simulink model "Model_15_11062020_3_Lev_Unbalance_SVM_AB21"  (R2021a)
settings: Solver=FixedStepAuto  StartTime=0.0  StopTime=0.03  FixedStep=Ts/10  MaxStep=1e-4  RelTol=1e-3
InitFcn:
  | Ts=1/(12000);
  | Ts_Control=Ts;
  | Ts_Power=Ts;
  | PulseDuration=5e-6;
  | Vrefpeak=399;
  | VDC=800;
  | R=1.4;
  | L=1e-4;
  | Freq = 120;
  | Rc= 0.00001;
  | C=220e-6;
  | Ld = 473e-6;
  | Lq = 1155e-6;
  | Fpm = 0.1383;
  | Rs = 0.036;
  | 
  | 
  | %%%%%Switch Characterization START%%%%%
  | T003_Thermal_Initialization;
  | T020_Characterizing_SKiM401MLI07E4_Simulink_Model_v1_0;
  | %%%%%Switch Characterization END%%%%%%
undefined symbols (not defined in the file or in its folder): Cond_Loss_Diode, Cond_Loss_IGBT, Page_Temp_C, Reverse_Rec_Diode, TurnoffIGBT, TurnonIGBT
libraries: spsMeanLib x35, simulink x28, spsMonostableLib x14, spsSampleandHoldLib x14, spsIGBTDiodeLib x12, spsDiodeLib x6, spsCurrentMeasurementLib x4, spsFirstOrderFilterLib x3, spsSeriesRLCBranchLib x3, spsVoltageMeasurementLib x3, pid_lib x2, spsAlphaBetaZerotoabcLib x1
(part 2 of 2)

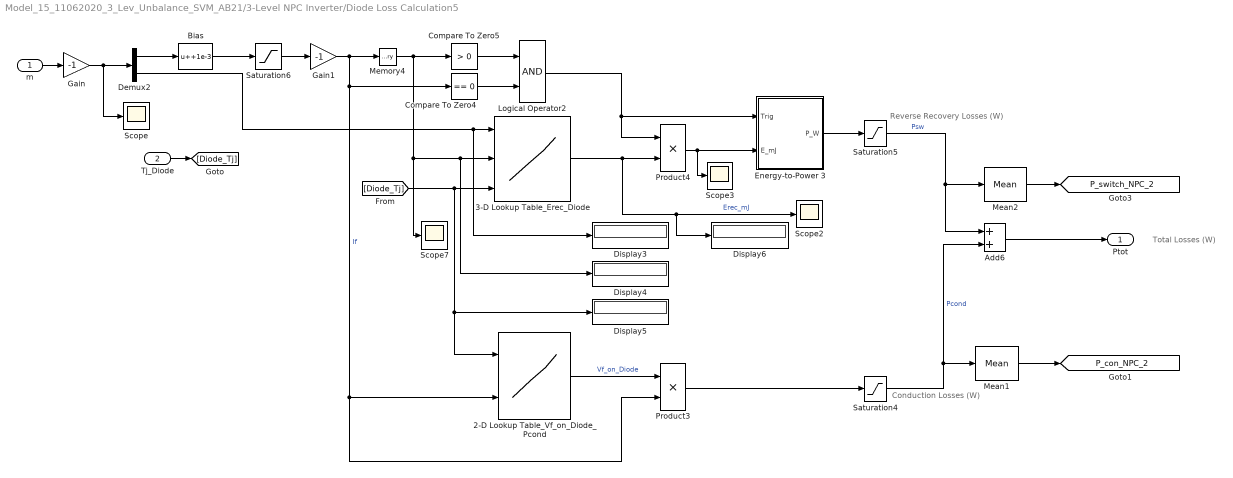
== system Model_15_11062020_3_Lev_Unbalance_SVM_AB21/3-Level NPC Inverter/Diode Loss Calculation5 ==
  note: Conduction Losses (W)
  note: Total Losses (W)
  note: Reverse Recovery Losses (W)
  m : Inport
  Tj_Diode : Inport  Port=2
  2-D Lookup Table_Vf_on_Diode_Pcond : Lookup_n-D  BreakpointsForDimension1=Cond_Loss_Diode.Tj  BreakpointsForDimension2=Cond_Loss_Diode.Ic  BreakpointsForDimension3=Page_Temp_C  Table=Cond_Loss_Diode.Vce  RndMeth=Simplest  InputSameDT=on
      settings: InputPortMap=u0,u1
  3-D Lookup Table_Erec_Diode : Lookup_n-D  NumberOfTableDimensions=3  BreakpointsForDimension1=Reverse_Rec_Diode.Vcc_Esw_Erec  BreakpointsForDimension2=Reverse_Rec_Diode.DIODE_If_Erec  BreakpointsForDimension3=Reverse_Rec_Diode.DIODE_Tj_Erec  Table=Reverse_Rec_Diode.Esw_Erec  RndMeth=Simplest  InputSameDT=on
      settings: InputPortMap=u0,u1,u2
  Add6 : Sum
  Bias : Bias  Bias=+1e-3
  Compare To Zero4 : simulink/Logic and Bit Operations/Compare To Zero  relop===  OutDataTypeStr=boolean
  Compare To Zero5 : simulink/Logic and Bit Operations/Compare To Zero  relop=>  OutDataTypeStr=boolean
  Demux2 : Demux  Outputs=2
  Display{3..6} (4 alike) : Display
  Energy-to-Power 3 : Subsystem  mask{PulseDuration=PulseDuration, Ts=Ts}
      mask prompts: PulseDuration "Pulse Duration (s):"; Ts "Sample time (s):"
  Gain : Gain  Gain=-1
  Gain1 : Gain  Gain=-1
  Logical Operator2 : Logic  AllPortsSameDT=off  OutDataTypeStr=float('double')
  Mean1 : spsMeanLib/Mean  Freq=Freq  Vinit=0  Ts=0
  Mean2 : spsMeanLib/Mean  Freq=Freq  Vinit=0  Ts=0
  Memory4 : Memory
  Product3 : Product  RndMeth=Zero
  Product4 : Product  RndMeth=Zero
  Saturation4 : Saturate  UpperLimit=inf  LowerLimit=0
  Saturation5 : Saturate  UpperLimit=inf  LowerLimit=0
  Saturation6 : Saturate  UpperLimit=0  LowerLimit=-1e6
  Scope{,2..3,7} (4 alike) : Scope
  Ptot : Outport  VectorParamsAs1DForOutWhenUnconnected=off
  tag scope: P_con_NPC_2=global, P_switch_NPC_2=global
  wires:
  Tj_Diode/1 -> [Diode_Tj]
  Compare To Zero4/1 -> Logical Operator2/2
  Logical Operator2/1 -> Energy-to-Power 3/1(Trig), Product4/1
  Gain1/1 -> Memory4/1, Product3/2, 2-D Lookup Table_Vf_on_Diode_Pcond/2, Compare To Zero4/1  "If"
  2-D Lookup Table_Vf_on_Diode_Pcond/1 -> Product3/1  "Vf_on_Diode"
  Demux2/1 -> Bias/1
  m/1 -> Gain/1
  Saturation6/1 -> Gain1/1
  Memory4/1 -> Compare To Zero5/1, Scope7/1, Display4/1, 3-D Lookup Table_Erec_Diode/2
  Demux2/2 -> Display3/1, 3-D Lookup Table_Erec_Diode/1
  Saturation4/1 -> Mean1/1, Add6/2  "Pcond"
  3-D Lookup Table_Erec_Diode/1 -> Display6/1, Scope2/1, Product4/2  "Erec_mJ"
  Saturation5/1 -> Mean2/1, Add6/1  "Psw"
  Product4/1 -> Scope3/1, Energy-to-Power 3/2(E_mJ)
  Energy-to-Power 3/1(P_W) -> Saturation5/1
  Product3/1 -> Saturation4/1
  [Diode_Tj] -> Display5/1, 2-D Lookup Table_Vf_on_Diode_Pcond/1, 3-D Lookup Table_Erec_Diode/3
  Compare To Zero5/1 -> Logical Operator2/1
  Add6/1 -> Ptot/1
  Bias/1 -> Saturation6/1
  Gain/1 -> Scope/1, Demux2/1
  Mean2/1 -> [P_switch_NPC_2]
  Mean1/1 -> [P_con_NPC_2]

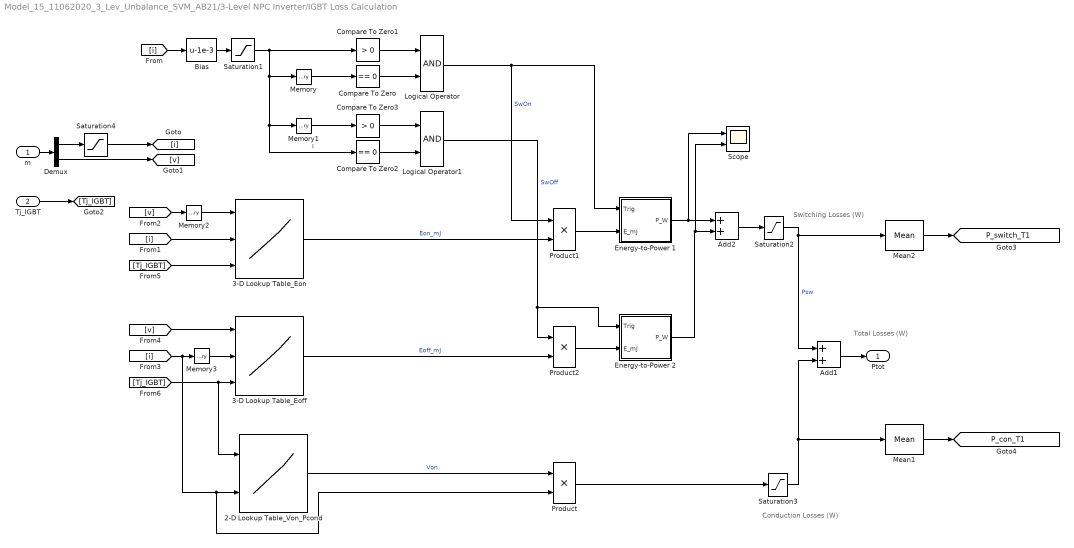
== system Model_15_11062020_3_Lev_Unbalance_SVM_AB21/3-Level NPC Inverter/IGBT Loss Calculation ==
  note: Switching Losses (W)
  note: Conduction Losses (W)
  note: Total Losses (W)
  m : Inport
  Tj_IGBT : Inport  Port=2
  2-D Lookup Table_Von_Pcond : Lookup_n-D  BreakpointsForDimension1=Cond_Loss_IGBT.Tj  BreakpointsForDimension2=Cond_Loss_IGBT.Ic  BreakpointsForDimension3=Page_Temp_C  Table=Cond_Loss_IGBT.Vce  RndMeth=Simplest  InputSameDT=on
      settings: InputPortMap=u0,u1
  3-D Lookup Table_Eoff : Lookup_n-D  NumberOfTableDimensions=3  BreakpointsForDimension1=TurnoffIGBT.Vcc_Esw_Off  BreakpointsForDimension2=TurnoffIGBT.Ic  BreakpointsForDimension3=TurnoffIGBT.Tj  Table=TurnoffIGBT.Esw_Off  RndMeth=Simplest  InputSameDT=on
      settings: InputPortMap=u0,u1,u2
  3-D Lookup Table_Eon : Lookup_n-D  NumberOfTableDimensions=3  BreakpointsForDimension1=TurnonIGBT.Vcc_Esw_On  BreakpointsForDimension2=TurnonIGBT.Ic  BreakpointsForDimension3=TurnonIGBT.Tj  Table=TurnonIGBT.Esw_On  RndMeth=Simplest  InputSameDT=on
      settings: InputPortMap=u0,u1,u2
  Add1 : Sum
  Add2 : Sum
  Bias : Bias  Bias=-1e-3
  Compare To Zero : simulink/Logic and Bit Operations/Compare To Zero  relop===  OutDataTypeStr=boolean
  Compare To Zero1 : simulink/Logic and Bit Operations/Compare To Zero  relop=>  OutDataTypeStr=boolean
  Compare To Zero2 : simulink/Logic and Bit Operations/Compare To Zero  relop===  OutDataTypeStr=boolean
  Compare To Zero3 : simulink/Logic and Bit Operations/Compare To Zero  relop=>  OutDataTypeStr=boolean
  Demux : Demux  Outputs=2
  Energy-to-Power 1 : Subsystem  mask{PulseDuration=PulseDuration, Ts=Ts}
      mask prompts: PulseDuration "Pulse Duration (s):"; Ts "Sample time (s):"
  Energy-to-Power 2 : Subsystem  mask{PulseDuration=PulseDuration, Ts=Ts}
      mask prompts: PulseDuration "Pulse Duration (s):"; Ts "Sample time (s):"
  Logical Operator : Logic  AllPortsSameDT=off  OutDataTypeStr=float('double')
  Logical Operator1 : Logic  AllPortsSameDT=off  OutDataTypeStr=float('double')
  Mean1 : spsMeanLib/Mean  Freq=Freq  Vinit=0  Ts=0
  Mean2 : spsMeanLib/Mean  Freq=Freq  Vinit=0  Ts=0
  Memory{,1..3} (4 alike) : Memory
  Product : Product  RndMeth=Zero
  Product1 : Product  RndMeth=Zero
  Product2 : Product  RndMeth=Zero
  Saturation1 : Saturate  UpperLimit=inf  LowerLimit=0
  Saturation2 : Saturate  UpperLimit=inf  LowerLimit=0
  Saturation3 : Saturate  UpperLimit=inf  LowerLimit=0
  Saturation4 : Saturate  UpperLimit=1e6  LowerLimit=0
  Scope : Scope  NumInputPorts=2
  Ptot : Outport  VectorParamsAs1DForOutWhenUnconnected=off
  tag scope: P_con_T1=global, P_switch_T1=global
  wires:
  Add1/1 -> Ptot/1
  Compare To Zero3/1 -> Logical Operator1/1
  Saturation1/1 -> Compare To Zero2/1, Memory1/1, Memory/1, Compare To Zero1/1  "I"
  Memory/1 -> Compare To Zero/1
  Compare To Zero2/1 -> Logical Operator1/2
  Compare To Zero1/1 -> Logical Operator/1
  [v] -> Memory2/1
  [i] -> 3-D Lookup Table_Eon/2
  Compare To Zero/1 -> Logical Operator/2
  Memory1/1 -> Compare To Zero3/1
  3-D Lookup Table_Eon/1 -> Product1/2  "Eon_mJ"
  Product/1 -> Saturation3/1
  3-D Lookup Table_Eoff/1 -> Product2/2  "Eoff_mJ"
  [i] -> Memory3/1, Product/2, 2-D Lookup Table_Von_Pcond/2
  Product1/1 -> Energy-to-Power 1/2(E_mJ)
  Logical Operator1/1 -> Product2/1, Energy-to-Power 2/1(Trig)  "SwOff"
  Energy-to-Power 2/1(P_W) -> Scope/2, Add2/2
  Logical Operator/1 -> Energy-to-Power 1/1(Trig), Product1/1  "SwOn"
  Energy-to-Power 1/1(P_W) -> Scope/1, Add2/1
  2-D Lookup Table_Von_Pcond/1 -> Product/1  "Von"
  [Tj_IGBT] -> 3-D Lookup Table_Eon/3
  [Tj_IGBT] -> 2-D Lookup Table_Von_Pcond/1, 3-D Lookup Table_Eoff/3
  Add2/1 -> Saturation2/1
  Product2/1 -> Energy-to-Power 2/2(E_mJ)
  [v] -> 3-D Lookup Table_Eoff/1
  Saturation2/1 -> Mean2/1, Add1/1  "Psw"
  m/1 -> Demux/1
  Demux/1 -> Saturation4/1
  Demux/2 -> [v]
  Tj_IGBT/1 -> [Tj_IGBT]
  Saturation4/1 -> [i]
  Memory3/1 -> 3-D Lookup Table_Eoff/2
  Mean1/1 -> [P_con_T1]
  Saturation3/1 -> Mean1/1, Add1/2
  Mean2/1 -> [P_switch_T1]
  [i] -> Bias/1
  Bias/1 -> Saturation1/1
  Memory2/1 -> 3-D Lookup Table_Eon/1

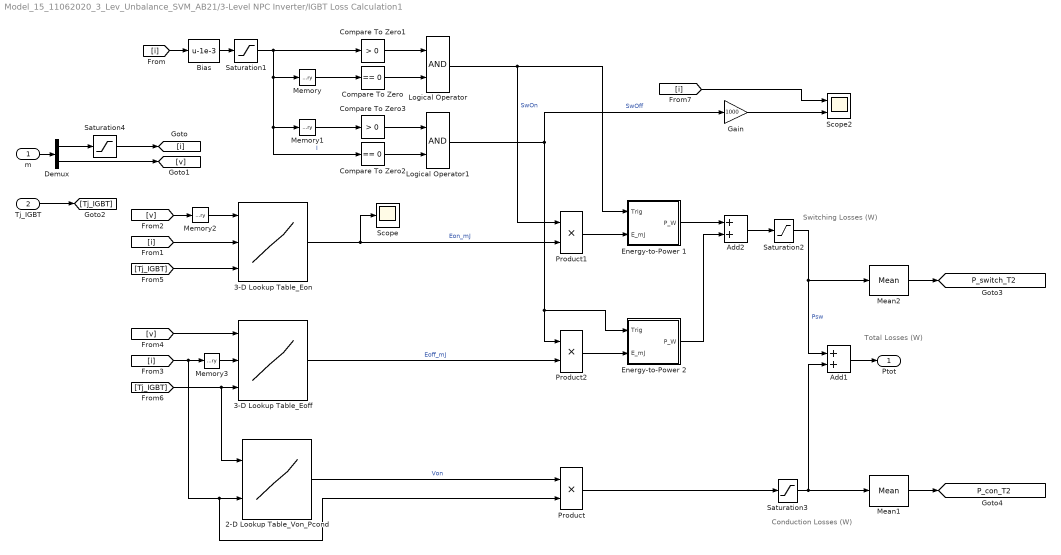
== system Model_15_11062020_3_Lev_Unbalance_SVM_AB21/3-Level NPC Inverter/IGBT Loss Calculation1 ==
  note: Switching Losses (W)
  note: Conduction Losses (W)
  note: Total Losses (W)
  m : Inport
  Tj_IGBT : Inport  Port=2
  2-D Lookup Table_Von_Pcond : Lookup_n-D  BreakpointsForDimension1=Cond_Loss_IGBT.Tj  BreakpointsForDimension2=Cond_Loss_IGBT.Ic  BreakpointsForDimension3=Page_Temp_C  Table=Cond_Loss_IGBT.Vce  RndMeth=Simplest  InputSameDT=on
      settings: InputPortMap=u0,u1
  3-D Lookup Table_Eoff : Lookup_n-D  NumberOfTableDimensions=3  BreakpointsForDimension1=TurnoffIGBT.Vcc_Esw_Off  BreakpointsForDimension2=TurnoffIGBT.Ic  BreakpointsForDimension3=TurnoffIGBT.Tj  Table=TurnoffIGBT.Esw_Off  RndMeth=Simplest  InputSameDT=on
      settings: InputPortMap=u0,u1,u2
  3-D Lookup Table_Eon : Lookup_n-D  NumberOfTableDimensions=3  BreakpointsForDimension1=TurnonIGBT.Vcc_Esw_On  BreakpointsForDimension2=TurnonIGBT.Ic  BreakpointsForDimension3=TurnonIGBT.Tj  Table=TurnonIGBT.Esw_On  RndMeth=Simplest  InputSameDT=on
      settings: InputPortMap=u0,u1,u2
  Add1 : Sum
  Add2 : Sum
  Bias : Bias  Bias=-1e-3
  Compare To Zero : simulink/Logic and Bit Operations/Compare To Zero  relop===  OutDataTypeStr=boolean
  Compare To Zero1 : simulink/Logic and Bit Operations/Compare To Zero  relop=>  OutDataTypeStr=boolean
  Compare To Zero2 : simulink/Logic and Bit Operations/Compare To Zero  relop===  OutDataTypeStr=boolean
  Compare To Zero3 : simulink/Logic and Bit Operations/Compare To Zero  relop=>  OutDataTypeStr=boolean
  Demux : Demux  Outputs=2
  Energy-to-Power 1 : Subsystem  mask{PulseDuration=PulseDuration, Ts=Ts}
      mask prompts: PulseDuration "Pulse Duration (s):"; Ts "Sample time (s):"
  Energy-to-Power 2 : Subsystem  mask{PulseDuration=PulseDuration, Ts=Ts}
      mask prompts: PulseDuration "Pulse Duration (s):"; Ts "Sample time (s):"
  Gain : Gain  Gain=1000
  Logical Operator : Logic  AllPortsSameDT=off  OutDataTypeStr=float('double')
  Logical Operator1 : Logic  AllPortsSameDT=off  OutDataTypeStr=float('double')
  Mean1 : spsMeanLib/Mean  Freq=Freq  Vinit=0  Ts=0
  Mean2 : spsMeanLib/Mean  Freq=Freq  Vinit=0  Ts=0
  Memory{,1..3} (4 alike) : Memory
  Product : Product  RndMeth=Zero
  Product1 : Product  RndMeth=Zero
  Product2 : Product  RndMeth=Zero
  Saturation1 : Saturate  UpperLimit=inf  LowerLimit=0
  Saturation2 : Saturate  UpperLimit=inf  LowerLimit=0
  Saturation3 : Saturate  UpperLimit=inf  LowerLimit=0
  Saturation4 : Saturate  UpperLimit=1e6  LowerLimit=0
  Scope : Scope
  Scope2 : Scope  NumInputPorts=2
  Ptot : Outport  VectorParamsAs1DForOutWhenUnconnected=off
  tag scope: P_con_T2=global, P_switch_T2=global
  wires:
  Add1/1 -> Ptot/1
  Compare To Zero3/1 -> Logical Operator1/1
  Saturation1/1 -> Compare To Zero2/1, Memory1/1, Memory/1, Compare To Zero1/1  "I"
  [v] -> Memory2/1
  Memory/1 -> Compare To Zero/1
  Compare To Zero2/1 -> Logical Operator1/2
  Compare To Zero1/1 -> Logical Operator/1
  Memory2/1 -> 3-D Lookup Table_Eon/1
  [i] -> 3-D Lookup Table_Eon/2
  Compare To Zero/1 -> Logical Operator/2
  Memory1/1 -> Compare To Zero3/1
  3-D Lookup Table_Eon/1 -> Scope/1, Product1/2  "Eon_mJ"
  Product/1 -> Saturation3/1
  Saturation3/1 -> Mean1/1, Add1/2
  3-D Lookup Table_Eoff/1 -> Product2/2  "Eoff_mJ"
  [i] -> Product/2, 2-D Lookup Table_Von_Pcond/2, Memory3/1
  Product1/1 -> Energy-to-Power 1/2(E_mJ)
  [i] -> Bias/1
  Logical Operator1/1 -> Gain/1, Product2/1, Energy-to-Power 2/1(Trig)  "SwOff"
  Energy-to-Power 2/1(P_W) -> Add2/2
  Logical Operator/1 -> Energy-to-Power 1/1(Trig), Product1/1  "SwOn"
  Energy-to-Power 1/1(P_W) -> Add2/1
  2-D Lookup Table_Von_Pcond/1 -> Product/1  "Von"
  [Tj_IGBT] -> 3-D Lookup Table_Eon/3
  [Tj_IGBT] -> 2-D Lookup Table_Von_Pcond/1, 3-D Lookup Table_Eoff/3
  Add2/1 -> Saturation2/1
  Product2/1 -> Energy-to-Power 2/2(E_mJ)
  [v] -> 3-D Lookup Table_Eoff/1
  Saturation2/1 -> Mean2/1, Add1/1  "Psw"
  m/1 -> Demux/1
  Demux/2 -> [v]
  Tj_IGBT/1 -> [Tj_IGBT]
  Saturation4/1 -> [i]
  Demux/1 -> Saturation4/1
  Memory3/1 -> 3-D Lookup Table_Eoff/2
  Mean1/1 -> [P_con_T2]
  Mean2/1 -> [P_switch_T2]
  [i] -> Scope2/1
  Gain/1 -> Scope2/2
  Bias/1 -> Saturation1/1

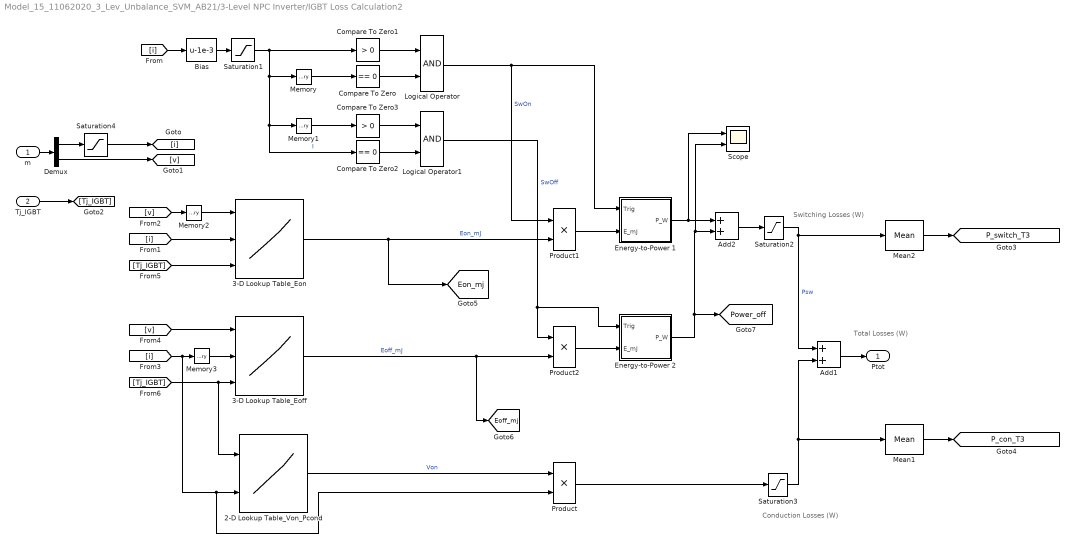
== system Model_15_11062020_3_Lev_Unbalance_SVM_AB21/3-Level NPC Inverter/IGBT Loss Calculation2 ==
  note: Switching Losses (W)
  note: Conduction Losses (W)
  note: Total Losses (W)
  m : Inport
  Tj_IGBT : Inport  Port=2
  2-D Lookup Table_Von_Pcond : Lookup_n-D  BreakpointsForDimension1=Cond_Loss_IGBT.Tj  BreakpointsForDimension2=Cond_Loss_IGBT.Ic  BreakpointsForDimension3=Page_Temp_C  Table=Cond_Loss_IGBT.Vce  RndMeth=Simplest  InputSameDT=on
      settings: InputPortMap=u0,u1
  3-D Lookup Table_Eoff : Lookup_n-D  NumberOfTableDimensions=3  BreakpointsForDimension1=TurnoffIGBT.Vcc_Esw_Off  BreakpointsForDimension2=TurnoffIGBT.Ic  BreakpointsForDimension3=TurnoffIGBT.Tj  Table=TurnoffIGBT.Esw_Off  RndMeth=Simplest  InputSameDT=on
      settings: InputPortMap=u0,u1,u2
  3-D Lookup Table_Eon : Lookup_n-D  NumberOfTableDimensions=3  BreakpointsForDimension1=TurnonIGBT.Vcc_Esw_On  BreakpointsForDimension2=TurnonIGBT.Ic  BreakpointsForDimension3=TurnonIGBT.Tj  Table=TurnonIGBT.Esw_On  RndMeth=Simplest  InputSameDT=on
      settings: InputPortMap=u0,u1,u2
  Add1 : Sum
  Add2 : Sum
  Bias : Bias  Bias=-1e-3
  Compare To Zero : simulink/Logic and Bit Operations/Compare To Zero  relop===  OutDataTypeStr=boolean
  Compare To Zero1 : simulink/Logic and Bit Operations/Compare To Zero  relop=>  OutDataTypeStr=boolean
  Compare To Zero2 : simulink/Logic and Bit Operations/Compare To Zero  relop===  OutDataTypeStr=boolean
  Compare To Zero3 : simulink/Logic and Bit Operations/Compare To Zero  relop=>  OutDataTypeStr=boolean
  Demux : Demux  Outputs=2
  Energy-to-Power 1 : Subsystem  mask{PulseDuration=PulseDuration, Ts=Ts}
      mask prompts: PulseDuration "Pulse Duration (s):"; Ts "Sample time (s):"
  Energy-to-Power 2 : Subsystem  mask{PulseDuration=PulseDuration, Ts=Ts}
      mask prompts: PulseDuration "Pulse Duration (s):"; Ts "Sample time (s):"
  Logical Operator : Logic  AllPortsSameDT=off  OutDataTypeStr=float('double')
  Logical Operator1 : Logic  AllPortsSameDT=off  OutDataTypeStr=float('double')
  Mean1 : spsMeanLib/Mean  Freq=Freq  Vinit=0  Ts=0
  Mean2 : spsMeanLib/Mean  Freq=Freq  Vinit=0  Ts=0
  Memory{,1..3} (4 alike) : Memory
  Product : Product  RndMeth=Zero
  Product1 : Product  RndMeth=Zero
  Product2 : Product  RndMeth=Zero
  Saturation1 : Saturate  UpperLimit=inf  LowerLimit=0
  Saturation2 : Saturate  UpperLimit=inf  LowerLimit=0
  Saturation3 : Saturate  UpperLimit=inf  LowerLimit=0
  Saturation4 : Saturate  UpperLimit=1e6  LowerLimit=0
  Scope : Scope  NumInputPorts=2
  Ptot : Outport  VectorParamsAs1DForOutWhenUnconnected=off
  tag scope: Eoff_mj=global, Eon_mj=global, P_con_T3=global, P_switch_T3=global, Power_off=global
  wires:
  Add1/1 -> Ptot/1
  Compare To Zero3/1 -> Logical Operator1/1
  Saturation1/1 -> Compare To Zero2/1, Memory1/1, Memory/1, Compare To Zero1/1  "I"
  Memory/1 -> Compare To Zero/1
  Compare To Zero2/1 -> Logical Operator1/2
  Compare To Zero1/1 -> Logical Operator/1
  [v] -> Memory2/1
  [i] -> 3-D Lookup Table_Eon/2
  Compare To Zero/1 -> Logical Operator/2
  Memory1/1 -> Compare To Zero3/1
  3-D Lookup Table_Eon/1 -> [Eon_mj], Product1/2  "Eon_mJ"
  Product/1 -> Saturation3/1
  3-D Lookup Table_Eoff/1 -> [Eoff_mj], Product2/2  "Eoff_mJ"
  [i] -> Memory3/1, Product/2, 2-D Lookup Table_Von_Pcond/2
  Product1/1 -> Energy-to-Power 1/2(E_mJ)
  Logical Operator1/1 -> Product2/1, Energy-to-Power 2/1(Trig)  "SwOff"
  Energy-to-Power 2/1(P_W) -> [Power_off], Scope/2, Add2/2
  Logical Operator/1 -> Energy-to-Power 1/1(Trig), Product1/1  "SwOn"
  Energy-to-Power 1/1(P_W) -> Scope/1, Add2/1
  2-D Lookup Table_Von_Pcond/1 -> Product/1  "Von"
  [Tj_IGBT] -> 3-D Lookup Table_Eon/3
  [Tj_IGBT] -> 2-D Lookup Table_Von_Pcond/1, 3-D Lookup Table_Eoff/3
  Add2/1 -> Saturation2/1
  Product2/1 -> Energy-to-Power 2/2(E_mJ)
  [v] -> 3-D Lookup Table_Eoff/1
  Saturation2/1 -> Mean2/1, Add1/1  "Psw"
  m/1 -> Demux/1
  Demux/1 -> Saturation4/1
  Demux/2 -> [v]
  Tj_IGBT/1 -> [Tj_IGBT]
  Saturation4/1 -> [i]
  Memory3/1 -> 3-D Lookup Table_Eoff/2
  Mean1/1 -> [P_con_T3]
  Saturation3/1 -> Mean1/1, Add1/2
  Mean2/1 -> [P_switch_T3]
  [i] -> Bias/1
  Bias/1 -> Saturation1/1
  Memory2/1 -> 3-D Lookup Table_Eon/1

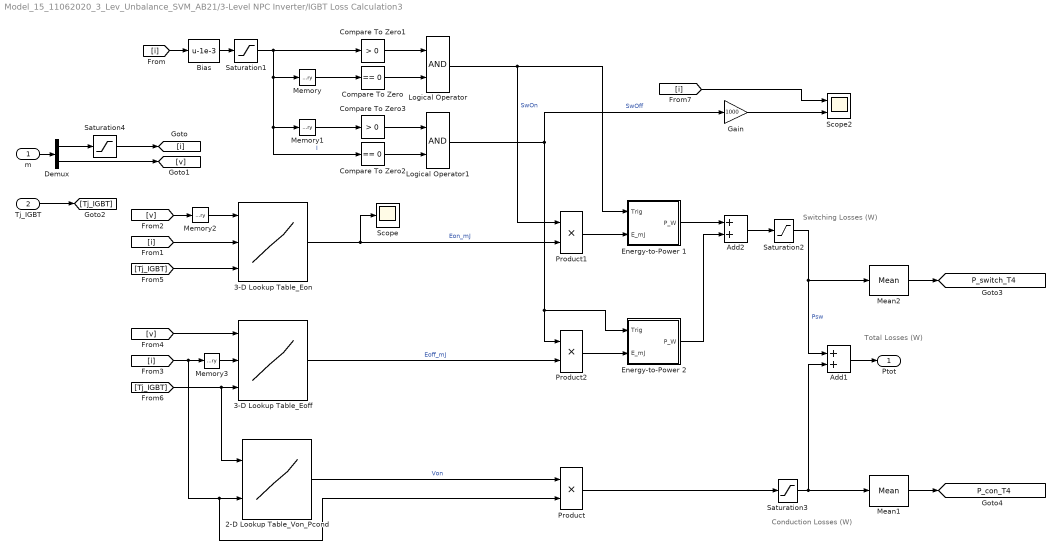
== system Model_15_11062020_3_Lev_Unbalance_SVM_AB21/3-Level NPC Inverter/IGBT Loss Calculation3 ==
  note: Switching Losses (W)
  note: Conduction Losses (W)
  note: Total Losses (W)
  m : Inport
  Tj_IGBT : Inport  Port=2
  2-D Lookup Table_Von_Pcond : Lookup_n-D  BreakpointsForDimension1=Cond_Loss_IGBT.Tj  BreakpointsForDimension2=Cond_Loss_IGBT.Ic  BreakpointsForDimension3=Page_Temp_C  Table=Cond_Loss_IGBT.Vce  RndMeth=Simplest  InputSameDT=on
      settings: InputPortMap=u0,u1
  3-D Lookup Table_Eoff : Lookup_n-D  NumberOfTableDimensions=3  BreakpointsForDimension1=TurnoffIGBT.Vcc_Esw_Off  BreakpointsForDimension2=TurnoffIGBT.Ic  BreakpointsForDimension3=TurnoffIGBT.Tj  Table=TurnoffIGBT.Esw_Off  RndMeth=Simplest  InputSameDT=on
      settings: InputPortMap=u0,u1,u2
  3-D Lookup Table_Eon : Lookup_n-D  NumberOfTableDimensions=3  BreakpointsForDimension1=TurnonIGBT.Vcc_Esw_On  BreakpointsForDimension2=TurnonIGBT.Ic  BreakpointsForDimension3=TurnonIGBT.Tj  Table=TurnonIGBT.Esw_On  RndMeth=Simplest  InputSameDT=on
      settings: InputPortMap=u0,u1,u2
  Add1 : Sum
  Add2 : Sum
  Bias : Bias  Bias=-1e-3
  Compare To Zero : simulink/Logic and Bit Operations/Compare To Zero  relop===  OutDataTypeStr=boolean
  Compare To Zero1 : simulink/Logic and Bit Operations/Compare To Zero  relop=>  OutDataTypeStr=boolean
  Compare To Zero2 : simulink/Logic and Bit Operations/Compare To Zero  relop===  OutDataTypeStr=boolean
  Compare To Zero3 : simulink/Logic and Bit Operations/Compare To Zero  relop=>  OutDataTypeStr=boolean
  Demux : Demux  Outputs=2
  Energy-to-Power 1 : Subsystem  mask{PulseDuration=PulseDuration, Ts=Ts}
      mask prompts: PulseDuration "Pulse Duration (s):"; Ts "Sample time (s):"
  Energy-to-Power 2 : Subsystem  mask{PulseDuration=PulseDuration, Ts=Ts}
      mask prompts: PulseDuration "Pulse Duration (s):"; Ts "Sample time (s):"
  Gain : Gain  Gain=1000
  Logical Operator : Logic  AllPortsSameDT=off  OutDataTypeStr=float('double')
  Logical Operator1 : Logic  AllPortsSameDT=off  OutDataTypeStr=float('double')
  Mean1 : spsMeanLib/Mean  Freq=Freq  Vinit=0  Ts=0
  Mean2 : spsMeanLib/Mean  Freq=Freq  Vinit=0  Ts=0
  Memory{,1..3} (4 alike) : Memory
  Product : Product  RndMeth=Zero
  Product1 : Product  RndMeth=Zero
  Product2 : Product  RndMeth=Zero
  Saturation1 : Saturate  UpperLimit=inf  LowerLimit=0
  Saturation2 : Saturate  UpperLimit=inf  LowerLimit=0
  Saturation3 : Saturate  UpperLimit=inf  LowerLimit=0
  Saturation4 : Saturate  UpperLimit=1e6  LowerLimit=0
  Scope : Scope
  Scope2 : Scope  NumInputPorts=2
  Ptot : Outport  VectorParamsAs1DForOutWhenUnconnected=off
  tag scope: P_con_T4=global, P_switch_T4=global
  wires:
  Add1/1 -> Ptot/1
  Compare To Zero3/1 -> Logical Operator1/1
  Saturation1/1 -> Compare To Zero2/1, Memory1/1, Memory/1, Compare To Zero1/1  "I"
  [v] -> Memory2/1
  Memory/1 -> Compare To Zero/1
  Compare To Zero2/1 -> Logical Operator1/2
  Compare To Zero1/1 -> Logical Operator/1
  Memory2/1 -> 3-D Lookup Table_Eon/1
  [i] -> 3-D Lookup Table_Eon/2
  Compare To Zero/1 -> Logical Operator/2
  Memory1/1 -> Compare To Zero3/1
  3-D Lookup Table_Eon/1 -> Scope/1, Product1/2  "Eon_mJ"
  Product/1 -> Saturation3/1
  Saturation3/1 -> Mean1/1, Add1/2
  3-D Lookup Table_Eoff/1 -> Product2/2  "Eoff_mJ"
  [i] -> Product/2, 2-D Lookup Table_Von_Pcond/2, Memory3/1
  Product1/1 -> Energy-to-Power 1/2(E_mJ)
  [i] -> Bias/1
  Logical Operator1/1 -> Gain/1, Product2/1, Energy-to-Power 2/1(Trig)  "SwOff"
  Energy-to-Power 2/1(P_W) -> Add2/2
  Logical Operator/1 -> Energy-to-Power 1/1(Trig), Product1/1  "SwOn"
  Energy-to-Power 1/1(P_W) -> Add2/1
  2-D Lookup Table_Von_Pcond/1 -> Product/1  "Von"
  [Tj_IGBT] -> 3-D Lookup Table_Eon/3
  [Tj_IGBT] -> 2-D Lookup Table_Von_Pcond/1, 3-D Lookup Table_Eoff/3
  Add2/1 -> Saturation2/1
  Product2/1 -> Energy-to-Power 2/2(E_mJ)
  [v] -> 3-D Lookup Table_Eoff/1
  Saturation2/1 -> Mean2/1, Add1/1  "Psw"
  m/1 -> Demux/1
  Demux/2 -> [v]
  Tj_IGBT/1 -> [Tj_IGBT]
  Saturation4/1 -> [i]
  Demux/1 -> Saturation4/1
  Memory3/1 -> 3-D Lookup Table_Eoff/2
  Mean1/1 -> [P_con_T4]
  Mean2/1 -> [P_switch_T4]
  [i] -> Scope2/1
  Gain/1 -> Scope2/2
  Bias/1 -> Saturation1/1

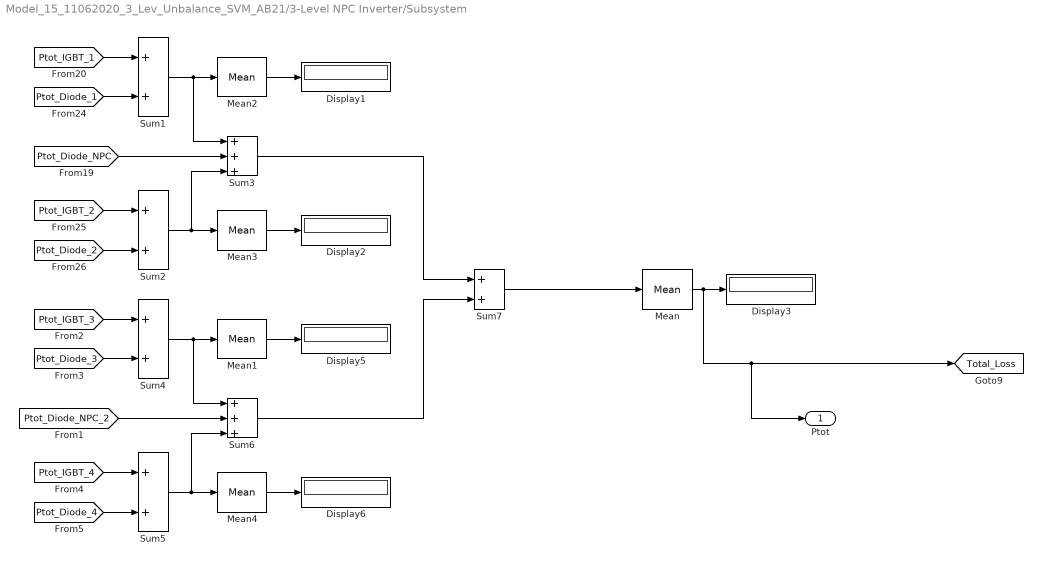
== system Model_15_11062020_3_Lev_Unbalance_SVM_AB21/3-Level NPC Inverter/Subsystem ==
  Display{1..3,5..6} (5 alike) : Display
  Mean{,1..4} (5 alike) : spsMeanLib/Mean  Freq=Freq  Vinit=0  Ts=0
  Sum{1..2,4..5,7} (5 alike) : Sum
  Sum3 : Sum  Inputs=+++
  Sum6 : Sum  Inputs=+++
  Ptot : Outport  VectorParamsAs1DForOutWhenUnconnected=off
  tag scope: Total_Loss=global
  wires:
  [Ptot_Diode_NPC] -> Sum3/2
  Mean2/1 -> Display1/1
  [Ptot_Diode_1] -> Sum1/2
  [Ptot_Diode_2] -> Sum2/2
  Mean/1 -> Ptot/1, [Total_Loss], Display3/1
  Sum1/1 -> Sum3/1, Mean2/1
  Sum2/1 -> Sum3/3, Mean3/1
  [Ptot_IGBT_1] -> Sum1/1
  [Ptot_IGBT_2] -> Sum2/1
  Mean3/1 -> Display2/1
  Sum5/1 -> Sum6/3, Mean4/1
  [Ptot_IGBT_4] -> Sum5/1
  [Ptot_IGBT_3] -> Sum4/1
  [Ptot_Diode_4] -> Sum5/2
  [Ptot_Diode_3] -> Sum4/2
  Mean1/1 -> Display5/1
  [Ptot_Diode_NPC_2] -> Sum6/2
  Mean4/1 -> Display6/1
  Sum4/1 -> Sum6/1, Mean1/1
  Sum6/1 -> Sum7/2
  Sum3/1 -> Sum7/1
  Sum7/1 -> Mean/1

== system Model_15_11062020_3_Lev_Unbalance_SVM_AB21/3-Level SVPWM/triangular gen ==
  Constant : Constant
  Gain : Gain  Gain=2
  Gain1 : Gain  Gain=2/(Ts)
  Integrator : Integrator
  Pulse Generator : DiscretePulseGenerator  PulseType=Time based  Period=Ts  PulseWidth=50
  Scope : Scope
  Sum : Sum  Inputs=|+-
  XTG : Outport
  wires:
  Gain1/1 -> Scope/1, XTG/1
  Integrator/1 -> Gain1/1
  Sum/1 -> Integrator/1
  Constant/1 -> Sum/2
  Gain/1 -> Sum/1
  Pulse Generator/1 -> Gain/1

== system Model_15_11062020_3_Lev_Unbalance_SVM_AB21/3-Level NPC Inverter/Diode Loss Calculation/Energy-to-Power 3 ==
  Trig : Inport
  E_mJ : Inport  Port=2
  Constant2 : Constant
  Constant3 : Constant  Value=0
  Monostable : spsMonostableLib/Monostable  EdgeDetect=Rising  PulseDuration=ceil(PulseDuration/Ts)*Ts  ic=0  Ts=Ts
      settings: SourceProductBaseCode=PS
  Product1 : Product  RndMeth=Zero
  Sample and Hold : spsSampleandHoldLib/Sample and Hold  ic=0  Ts=Ts
      settings: SourceProductBaseCode=PS
  Switch1 : Switch  Criteria=u2 ~= 0
  gain : Gain  Gain=1e-3/(ceil(PulseDuration/Ts)*Ts)
  P_W : Outport  VectorParamsAs1DForOutWhenUnconnected=off
  wires:
  Product1/1 -> P_W/1
  Sample and Hold/1 -> Product1/1
  gain/1 -> Sample and Hold/1
  Trig/1 -> Sample and Hold/2, Monostable/1
  E_mJ/1 -> gain/1
  Monostable/1 -> Switch1/2
  Constant2/1 -> Switch1/1
  Constant3/1 -> Switch1/3
  Switch1/1 -> Product1/2

== system Model_15_11062020_3_Lev_Unbalance_SVM_AB21/3-Level NPC Inverter/Diode Loss Calculation1/Energy-to-Power 3 ==
  Trig : Inport
  E_mJ : Inport  Port=2
  Constant2 : Constant
  Constant3 : Constant  Value=0
  Monostable : spsMonostableLib/Monostable  EdgeDetect=Rising  PulseDuration=ceil(PulseDuration/Ts)*Ts  ic=0  Ts=Ts
      settings: SourceProductBaseCode=PS
  Product1 : Product  RndMeth=Zero
  Sample and Hold : spsSampleandHoldLib/Sample and Hold  ic=0  Ts=Ts
      settings: SourceProductBaseCode=PS
  Switch1 : Switch  Criteria=u2 ~= 0
  gain : Gain  Gain=1e-3/(ceil(PulseDuration/Ts)*Ts)
  P_W : Outport  VectorParamsAs1DForOutWhenUnconnected=off
  wires:
  Product1/1 -> P_W/1
  Sample and Hold/1 -> Product1/1
  gain/1 -> Sample and Hold/1
  Trig/1 -> Sample and Hold/2, Monostable/1
  E_mJ/1 -> gain/1
  Monostable/1 -> Switch1/2
  Constant2/1 -> Switch1/1
  Constant3/1 -> Switch1/3
  Switch1/1 -> Product1/2

== system Model_15_11062020_3_Lev_Unbalance_SVM_AB21/3-Level NPC Inverter/Diode Loss Calculation2/Energy-to-Power 3 ==
  Trig : Inport
  E_mJ : Inport  Port=2
  Constant2 : Constant
  Constant3 : Constant  Value=0
  Monostable : spsMonostableLib/Monostable  EdgeDetect=Rising  PulseDuration=ceil(PulseDuration/Ts)*Ts  ic=0  Ts=Ts
      settings: SourceProductBaseCode=PS
  Product1 : Product  RndMeth=Zero
  Sample and Hold : spsSampleandHoldLib/Sample and Hold  ic=0  Ts=Ts
      settings: SourceProductBaseCode=PS
  Switch1 : Switch  Criteria=u2 ~= 0
  gain : Gain  Gain=1e-3/(ceil(PulseDuration/Ts)*Ts)
  P_W : Outport  VectorParamsAs1DForOutWhenUnconnected=off
  wires:
  Product1/1 -> P_W/1
  Sample and Hold/1 -> Product1/1
  gain/1 -> Sample and Hold/1
  Trig/1 -> Sample and Hold/2, Monostable/1
  E_mJ/1 -> gain/1
  Monostable/1 -> Switch1/2
  Constant2/1 -> Switch1/1
  Constant3/1 -> Switch1/3
  Switch1/1 -> Product1/2

== system Model_15_11062020_3_Lev_Unbalance_SVM_AB21/3-Level NPC Inverter/Diode Loss Calculation3/Energy-to-Power 3 ==
  Trig : Inport
  E_mJ : Inport  Port=2
  Constant2 : Constant
  Constant3 : Constant  Value=0
  Monostable : spsMonostableLib/Monostable  EdgeDetect=Rising  PulseDuration=ceil(PulseDuration/Ts)*Ts  ic=0  Ts=Ts
      settings: SourceProductBaseCode=PS
  Product1 : Product  RndMeth=Zero
  Sample and Hold : spsSampleandHoldLib/Sample and Hold  ic=0  Ts=Ts
      settings: SourceProductBaseCode=PS
  Switch1 : Switch  Criteria=u2 ~= 0
  gain : Gain  Gain=1e-3/(ceil(PulseDuration/Ts)*Ts)
  P_W : Outport  VectorParamsAs1DForOutWhenUnconnected=off
  wires:
  Product1/1 -> P_W/1
  Sample and Hold/1 -> Product1/1
  gain/1 -> Sample and Hold/1
  Trig/1 -> Sample and Hold/2, Monostable/1
  E_mJ/1 -> gain/1
  Monostable/1 -> Switch1/2
  Constant2/1 -> Switch1/1
  Constant3/1 -> Switch1/3
  Switch1/1 -> Product1/2

== system Model_15_11062020_3_Lev_Unbalance_SVM_AB21/3-Level NPC Inverter/Diode Loss Calculation4/Energy-to-Power 3 ==
  Trig : Inport
  E_mJ : Inport  Port=2
  Constant2 : Constant
  Constant3 : Constant  Value=0
  Monostable : spsMonostableLib/Monostable  EdgeDetect=Rising  PulseDuration=ceil(PulseDuration/Ts)*Ts  ic=0  Ts=Ts
      settings: SourceProductBaseCode=PS
  Product1 : Product  RndMeth=Zero
  Sample and Hold : spsSampleandHoldLib/Sample and Hold  ic=0  Ts=Ts
      settings: SourceProductBaseCode=PS
  Switch1 : Switch  Criteria=u2 ~= 0
  gain : Gain  Gain=1e-3/(ceil(PulseDuration/Ts)*Ts)
  P_W : Outport  VectorParamsAs1DForOutWhenUnconnected=off
  wires:
  Switch1/1 -> Product1/2
  Constant3/1 -> Switch1/3
  Constant2/1 -> Switch1/1
  Monostable/1 -> Switch1/2
  E_mJ/1 -> gain/1
  Trig/1 -> Monostable/1, Sample and Hold/2
  gain/1 -> Sample and Hold/1
  Sample and Hold/1 -> Product1/1
  Product1/1 -> P_W/1

== system Model_15_11062020_3_Lev_Unbalance_SVM_AB21/3-Level NPC Inverter/Diode Loss Calculation5/Energy-to-Power 3 ==
  Trig : Inport
  E_mJ : Inport  Port=2
  Constant2 : Constant
  Constant3 : Constant  Value=0
  Monostable : spsMonostableLib/Monostable  EdgeDetect=Rising  PulseDuration=ceil(PulseDuration/Ts)*Ts  ic=0  Ts=Ts
      settings: SourceProductBaseCode=PS
  Product1 : Product  RndMeth=Zero
  Sample and Hold : spsSampleandHoldLib/Sample and Hold  ic=0  Ts=Ts
      settings: SourceProductBaseCode=PS
  Switch1 : Switch  Criteria=u2 ~= 0
  gain : Gain  Gain=1e-3/(ceil(PulseDuration/Ts)*Ts)
  P_W : Outport  VectorParamsAs1DForOutWhenUnconnected=off
  wires:
  Switch1/1 -> Product1/2
  Constant3/1 -> Switch1/3
  Constant2/1 -> Switch1/1
  Monostable/1 -> Switch1/2
  E_mJ/1 -> gain/1
  Trig/1 -> Monostable/1, Sample and Hold/2
  gain/1 -> Sample and Hold/1
  Sample and Hold/1 -> Product1/1
  Product1/1 -> P_W/1

== system Model_15_11062020_3_Lev_Unbalance_SVM_AB21/3-Level NPC Inverter/IGBT Loss Calculation/Energy-to-Power 1 ==
  Trig : Inport
  E_mJ : Inport  Port=2
  Constant2 : Constant
  Constant3 : Constant  Value=0
  Monostable : spsMonostableLib/Monostable  EdgeDetect=Rising  PulseDuration=ceil(PulseDuration/Ts)*Ts  ic=0  Ts=Ts
      settings: SourceProductBaseCode=PS
  Product1 : Product  RndMeth=Zero
  Sample and Hold : spsSampleandHoldLib/Sample and Hold  ic=0  Ts=Ts
      settings: SourceProductBaseCode=PS
  Switch1 : Switch  Criteria=u2 ~= 0
  gain : Gain  Gain=1e-3/(ceil(PulseDuration/Ts)*Ts)
  P_W : Outport  VectorParamsAs1DForOutWhenUnconnected=off
  wires:
  Product1/1 -> P_W/1
  Sample and Hold/1 -> Product1/1
  gain/1 -> Sample and Hold/1
  Trig/1 -> Sample and Hold/2, Monostable/1
  E_mJ/1 -> gain/1
  Monostable/1 -> Switch1/2
  Constant2/1 -> Switch1/1
  Constant3/1 -> Switch1/3
  Switch1/1 -> Product1/2

== system Model_15_11062020_3_Lev_Unbalance_SVM_AB21/3-Level NPC Inverter/IGBT Loss Calculation/Energy-to-Power 2 ==
  Trig : Inport
  E_mJ : Inport  Port=2
  Constant2 : Constant
  Constant3 : Constant  Value=0
  Monostable : spsMonostableLib/Monostable  EdgeDetect=Rising  PulseDuration=ceil(PulseDuration/Ts)*Ts  ic=0  Ts=Ts
      settings: SourceProductBaseCode=PS
  Product1 : Product  RndMeth=Zero
  Sample and Hold : spsSampleandHoldLib/Sample and Hold  ic=0  Ts=Ts
      settings: SourceProductBaseCode=PS
  Switch1 : Switch  Criteria=u2 ~= 0
  gain : Gain  Gain=1e-3/(ceil(PulseDuration/Ts)*Ts)
  P_W : Outport  VectorParamsAs1DForOutWhenUnconnected=off
  wires:
  Product1/1 -> P_W/1
  Sample and Hold/1 -> Product1/1
  gain/1 -> Sample and Hold/1
  Trig/1 -> Sample and Hold/2, Monostable/1
  E_mJ/1 -> gain/1
  Monostable/1 -> Switch1/2
  Constant2/1 -> Switch1/1
  Constant3/1 -> Switch1/3
  Switch1/1 -> Product1/2

== system Model_15_11062020_3_Lev_Unbalance_SVM_AB21/3-Level NPC Inverter/IGBT Loss Calculation1/Energy-to-Power 1 ==
  Trig : Inport
  E_mJ : Inport  Port=2
  Constant2 : Constant
  Constant3 : Constant  Value=0
  Monostable : spsMonostableLib/Monostable  EdgeDetect=Rising  PulseDuration=ceil(PulseDuration/Ts)*Ts  ic=0  Ts=Ts
      settings: SourceProductBaseCode=PS
  Product1 : Product  RndMeth=Zero
  Sample and Hold : spsSampleandHoldLib/Sample and Hold  ic=0  Ts=Ts
      settings: SourceProductBaseCode=PS
  Switch1 : Switch  Criteria=u2 ~= 0
  gain : Gain  Gain=1e-3/(ceil(PulseDuration/Ts)*Ts)
  P_W : Outport  VectorParamsAs1DForOutWhenUnconnected=off
  wires:
  Product1/1 -> P_W/1
  Sample and Hold/1 -> Product1/1
  gain/1 -> Sample and Hold/1
  Trig/1 -> Sample and Hold/2, Monostable/1
  E_mJ/1 -> gain/1
  Monostable/1 -> Switch1/2
  Constant2/1 -> Switch1/1
  Constant3/1 -> Switch1/3
  Switch1/1 -> Product1/2

== system Model_15_11062020_3_Lev_Unbalance_SVM_AB21/3-Level NPC Inverter/IGBT Loss Calculation1/Energy-to-Power 2 ==
  Trig : Inport
  E_mJ : Inport  Port=2
  Constant2 : Constant
  Constant3 : Constant  Value=0
  Monostable : spsMonostableLib/Monostable  EdgeDetect=Rising  PulseDuration=ceil(PulseDuration/Ts)*Ts  ic=0  Ts=Ts
      settings: SourceProductBaseCode=PS
  Product1 : Product  RndMeth=Zero
  Sample and Hold : spsSampleandHoldLib/Sample and Hold  ic=0  Ts=Ts
      settings: SourceProductBaseCode=PS
  Switch1 : Switch  Criteria=u2 ~= 0
  gain : Gain  Gain=1e-3/(ceil(PulseDuration/Ts)*Ts)
  P_W : Outport  VectorParamsAs1DForOutWhenUnconnected=off
  wires:
  Product1/1 -> P_W/1
  Sample and Hold/1 -> Product1/1
  gain/1 -> Sample and Hold/1
  Trig/1 -> Sample and Hold/2, Monostable/1
  E_mJ/1 -> gain/1
  Monostable/1 -> Switch1/2
  Constant2/1 -> Switch1/1
  Constant3/1 -> Switch1/3
  Switch1/1 -> Product1/2

== system Model_15_11062020_3_Lev_Unbalance_SVM_AB21/3-Level NPC Inverter/IGBT Loss Calculation2/Energy-to-Power 1 ==
  Trig : Inport
  E_mJ : Inport  Port=2
  Constant2 : Constant
  Constant3 : Constant  Value=0
  Monostable : spsMonostableLib/Monostable  EdgeDetect=Rising  PulseDuration=ceil(PulseDuration/Ts)*Ts  ic=0  Ts=Ts
      settings: SourceProductBaseCode=PS
  Product1 : Product  RndMeth=Zero
  Sample and Hold : spsSampleandHoldLib/Sample and Hold  ic=0  Ts=Ts
      settings: SourceProductBaseCode=PS
  Switch1 : Switch  Criteria=u2 ~= 0
  gain : Gain  Gain=1e-3/(ceil(PulseDuration/Ts)*Ts)
  P_W : Outport  VectorParamsAs1DForOutWhenUnconnected=off
  wires:
  Product1/1 -> P_W/1
  Sample and Hold/1 -> Product1/1
  gain/1 -> Sample and Hold/1
  Trig/1 -> Sample and Hold/2, Monostable/1
  E_mJ/1 -> gain/1
  Monostable/1 -> Switch1/2
  Constant2/1 -> Switch1/1
  Constant3/1 -> Switch1/3
  Switch1/1 -> Product1/2

== system Model_15_11062020_3_Lev_Unbalance_SVM_AB21/3-Level NPC Inverter/IGBT Loss Calculation2/Energy-to-Power 2 ==
  Trig : Inport
  E_mJ : Inport  Port=2
  Constant2 : Constant
  Constant3 : Constant  Value=0
  Monostable : spsMonostableLib/Monostable  EdgeDetect=Rising  PulseDuration=ceil(PulseDuration/Ts)*Ts  ic=0  Ts=Ts
      settings: SourceProductBaseCode=PS
  Product1 : Product  RndMeth=Zero
  Sample and Hold : spsSampleandHoldLib/Sample and Hold  ic=0  Ts=Ts
      settings: SourceProductBaseCode=PS
  Switch1 : Switch  Criteria=u2 ~= 0
  gain : Gain  Gain=1e-3/(ceil(PulseDuration/Ts)*Ts)
  P_W : Outport  VectorParamsAs1DForOutWhenUnconnected=off
  wires:
  Product1/1 -> P_W/1
  Sample and Hold/1 -> Product1/1
  gain/1 -> Sample and Hold/1
  Trig/1 -> Sample and Hold/2, Monostable/1
  E_mJ/1 -> gain/1
  Monostable/1 -> Switch1/2
  Constant2/1 -> Switch1/1
  Constant3/1 -> Switch1/3
  Switch1/1 -> Product1/2

== system Model_15_11062020_3_Lev_Unbalance_SVM_AB21/3-Level NPC Inverter/IGBT Loss Calculation3/Energy-to-Power 1 ==
  Trig : Inport
  E_mJ : Inport  Port=2
  Constant2 : Constant
  Constant3 : Constant  Value=0
  Monostable : spsMonostableLib/Monostable  EdgeDetect=Rising  PulseDuration=ceil(PulseDuration/Ts)*Ts  ic=0  Ts=Ts
      settings: SourceProductBaseCode=PS
  Product1 : Product  RndMeth=Zero
  Sample and Hold : spsSampleandHoldLib/Sample and Hold  ic=0  Ts=Ts
      settings: SourceProductBaseCode=PS
  Switch1 : Switch  Criteria=u2 ~= 0
  gain : Gain  Gain=1e-3/(ceil(PulseDuration/Ts)*Ts)
  P_W : Outport  VectorParamsAs1DForOutWhenUnconnected=off
  wires:
  Product1/1 -> P_W/1
  Sample and Hold/1 -> Product1/1
  gain/1 -> Sample and Hold/1
  Trig/1 -> Sample and Hold/2, Monostable/1
  E_mJ/1 -> gain/1
  Monostable/1 -> Switch1/2
  Constant2/1 -> Switch1/1
  Constant3/1 -> Switch1/3
  Switch1/1 -> Product1/2

== system Model_15_11062020_3_Lev_Unbalance_SVM_AB21/3-Level NPC Inverter/IGBT Loss Calculation3/Energy-to-Power 2 ==
  Trig : Inport
  E_mJ : Inport  Port=2
  Constant2 : Constant
  Constant3 : Constant  Value=0
  Monostable : spsMonostableLib/Monostable  EdgeDetect=Rising  PulseDuration=ceil(PulseDuration/Ts)*Ts  ic=0  Ts=Ts
      settings: SourceProductBaseCode=PS
  Product1 : Product  RndMeth=Zero
  Sample and Hold : spsSampleandHoldLib/Sample and Hold  ic=0  Ts=Ts
      settings: SourceProductBaseCode=PS
  Switch1 : Switch  Criteria=u2 ~= 0
  gain : Gain  Gain=1e-3/(ceil(PulseDuration/Ts)*Ts)
  P_W : Outport  VectorParamsAs1DForOutWhenUnconnected=off
  wires:
  Product1/1 -> P_W/1
  Sample and Hold/1 -> Product1/1
  gain/1 -> Sample and Hold/1
  Trig/1 -> Sample and Hold/2, Monostable/1
  E_mJ/1 -> gain/1
  Monostable/1 -> Switch1/2
  Constant2/1 -> Switch1/1
  Constant3/1 -> Switch1/3
  Switch1/1 -> Product1/2

== matlab function Model_15_11062020_3_Lev_Unbalance_SVM_AB21/3-Level SVPWM/Sector Angle ==
  data: theta input; phi output; sector input
function phi= fcn(theta,sector)
phi=0;
if(sector==1)
    phi=theta;
end
if(sector==2)
    phi=theta-pi/3;
end
if(sector==3)
    phi=theta-2*pi/3;
end
if(sector==6)
    phi=theta+pi/3;
end
if(sector==5)
    phi=theta+2*pi/3;
end
if(sector==4)
    phi=theta+pi;
end
end

== matlab function Model_15_11062020_3_Lev_Unbalance_SVM_AB21/3-Level SVPWM/Region Selection ==
  data: Vref input; region output; phi input; Vdc input
function region = fcn(Vref,phi,Vdc)
region=0;
m=0;
m1=0;
m2=0;
m=Vref/(2/3*Vdc);
m1=m*2/sqrt(3)*sin(pi/3-phi);
m2=m*2/sqrt(3)*sin(phi);


if (m1<0.5)&&(m2<0.5)&&(m1+m2<0.5)
    region=1;
end
if (m1<0.5)&&(m2<0.5)&&(m1+m2>0.5)
    region=2;
end
if (m1>0.5)
    region=4;
end
if(m2>0.5)
    region=3;
end
end

== matlab function Model_15_11062020_3_Lev_Unbalance_SVM_AB21/3-Level SVPWM/Vector Switching ==
  data: Vref input; region input; Ta output; phi input; Vdc input; Ts input; Tb output; Tc output
function [Ta,Tb,Tc]= fcn(Vref,region, phi,Vdc,Ts)
Ta=0;
Tb=0;
Tc=0;
m=0;
k=0;
m=Vref/(2/3*Vdc);
k=2/sqrt(3)*m*Ts;
if(region==1)
    Ta=2*k*sin(pi/3-phi);
    Tb=Ts-2*k*sin(pi/3+phi);
    Tc=2*k*sin(phi);
end
if(region==2)
     Ta=Ts-2*k*sin(phi);
     Tb=2*k*sin(pi/3+phi)-Ts;
     Tc=Ts-2*k*sin(pi/3-phi);
end
if(region==3)
    Ta=2*k*sin(phi)-Ts;
    Tb=2*k*sin(pi/3-phi);
    Tc=2*Ts-2*k*sin(pi/3+phi);
end
if(region==4)
    Ta=2*Ts-2*k*sin(pi/3+phi);
    Tb=2*k*sin(phi);
    Tc=2*k*sin(pi/3-phi)-Ts;
end
end

== matlab function Model_15_11062020_3_Lev_Unbalance_SVM_AB21/3-Level SVPWM/Region Switching ==
  data: region input; Ta input; S1A output; Tb input; Tc input; Ts input; S2A output; S1B output; S2B output; S1C output; S2C output
function [S1A,S2A,S1B,S2B,S1C,S2C]= fcn(region,Ta,Tb,Tc,Ts)
S1A=0;
S2A=0;
S1B=0;
S2B=0;
S1C=0;
S2C=0;
if(region==1)
    S1A=Tc/4+Ta/4;
    S2A=Ts/2;
    S1B=Tc/4;
    S2B=Ts/2-Ta/4;
    S1C=0;
    S2C=Ts/2-Ta/4-Tc/4;
end
if(region==2)
    S1A=Tc/4+Ta/4+Tb/4;
    S2A=Ts/2;
    S1B=Tc/4;
    S2B=Ts/2-Ta/4;
    S1C=0;
    S2C=Ta/4+Tc/4;
end
if(region==3)
    S1A=Ts/2-Tc/4;
    S2A=Ts/2;
    S1B=Tc/4+Ta/2;
    S2B=Ts/2;
    S1C=0;
    S2C=Tc/4;
end
if(region==4)
    S1A=Ts/2-Ta/4;
    S2A=Ts/2;
    S1B=0;
    S2B=Ta/4+Tb/2;
    S1C=0;
    S2C=Ta/4;
end
end

== matlab function Model_15_11062020_3_Lev_Unbalance_SVM_AB21/3-Level SVPWM/Sector Switching ==
  data: sector input; S1A input; g1a output; S2A input; S1B input; S2B input; S1C input; S2C input; Ts input; g2a output; g1b output; g2b output; g1c output; g2c output
function [g1a,g2a,g1b,g2b,g1c,g2c] = fcn(sector,S1A,S2A,S1B,S2B,S1C,S2C,Ts)
g1a=0;
g2a=0;
g1b=0;
g2b=0;
g1c=0;
g2c=0;
if(sector==1)
   g1a=S1A;
   g2a=S2A;
   g1b=S1B;
   g2b=S2B;
   g1c=S1C;
   g2c=S2C;
end
if(sector==2)
    g1a=Ts/2-S2B;
    g2a=Ts/2-S1B;
    g1b=Ts/2-S2C;
    g2b=Ts/2-S1C;
    g1c=Ts/2-S2A;
    g2c=Ts/2-S1A;
end
if(sector==3)
    g1a=S1C;
   g2a=S2C;
   g1b=S1A;
   g2b=S2A;
   g1c=S1B;
   g2c=S2B;
end
if(sector==4)
    g1a=Ts/2-S2A;
    g2a=Ts/2-S1A;
    g1b=Ts/2-S2B;
    g2b=Ts/2-S1B;
    g1c=Ts/2-S2C;
    g2c=Ts/2-S1C;
end
if(sector==5)
    g1a=S1B;
   g2a=S2B;
   g1b=S1C;
   g2b=S2C;
   g1c=S1A;
   g2c=S2A;
end
if(sector==6)
    g1a=Ts/2-S2C;
    g2a=Ts/2-S1C;
    g1b=Ts/2-S2A;
    g2b=Ts/2-S1A;
    g1c=Ts/2-S2B;
    g2c=Ts/2-S1B;
end
end

== matlab function Model_15_11062020_3_Lev_Unbalance_SVM_AB21/3-Level SVPWM/Sector Selection ==
  data: theta input; sector output
function sector = fcn(theta)
sector=0;
if (theta>=0)&&(theta<pi/3)
    sector=1;
end
if (theta>=pi/3)&&(theta<2*pi/3)
    sector=2;
end
if (theta>=2*pi/3)&&(theta<pi)
    sector=3;
end
if (theta>=-pi)&&(theta<-2*pi/3)
    sector=4;
end
if (theta>=-2*pi/3)&&(theta<-pi/3)
    sector=5;
end
if (theta>=-pi/3)&&(theta<0)
    sector=6;
end
end
